simulink library "mbd_s32k11_ec_toolbox"  (Simulink 9.0)
settings: Solver=FixedStepDiscrete  StartTime=0.0  StopTime=10.0  FixedStep=0.1  RelTol=1e-3
InitFcn:
  | mbd_s32k11_consistency_checks(bdroot(gcs));
(part 1 of 2)
settings Model: Creator=evarshavskaya  LastModifiedBy=nxf30742

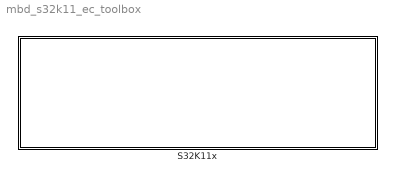
== system mbd_s32k11_ec_toolbox ==
  S32K11x : Subsystem

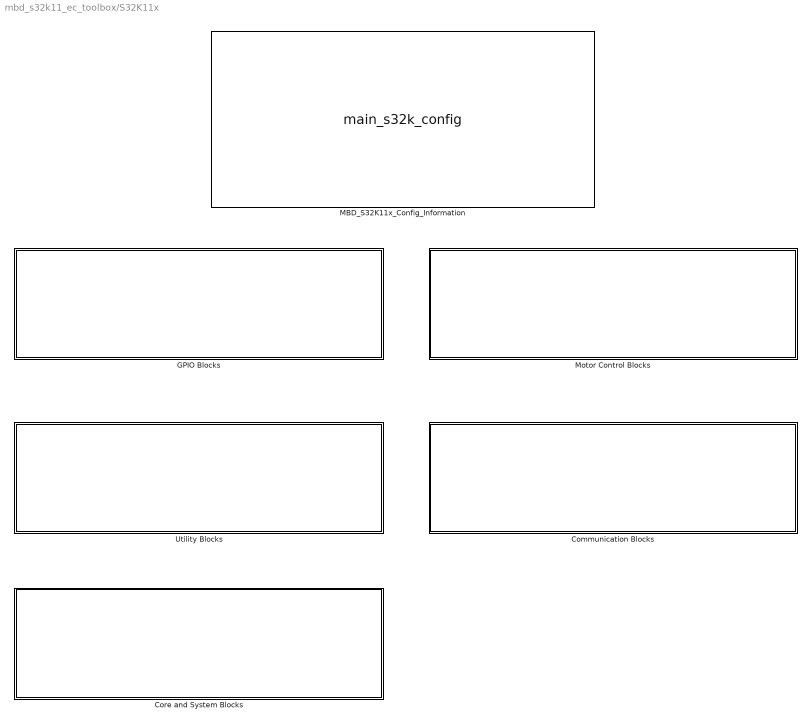
== system mbd_s32k11_ec_toolbox/S32K11x ==
  Communication Blocks : Subsystem
  Core and System Blocks : Subsystem
  GPIO Blocks : Subsystem
  MBD_S32K11x_Config_Information : S-Function  LoadFcn=|  InitFcn=|  FunctionName=main_s32k_config  SFunctionDeploymentMode=off  EnableBusSupport=off  mask(MBDTBX_EC_S32K11){disp_str=|, config_params=[], mcu_target_name=S32K116, mcu_target_package=48-LQFP, mcu_target_sram_size=17KB, mcu_system_clock_freq=40, mcu_xtal_freq=External 40, mcu_steptick_timer=LPIT Channel 0, mcu_steptick_prio=3, ds_import_enable=on, target_compiler=GCC, target_memory=FLASH, gcc_target_compile_opts=-mthumb -O1 -g -gstrict-dwarf, gcc_target_assemble_opts=-mthumb -g, gcc_target_link_opts=-mthumb, gcc_target_lib_opts=, gcc_target_default_lcf=on, gcc_target_user_lcf=S32K116_17_flash.ld, ghs_target_compile_opts=-thumb -fsingle -Ogeneral -Wundef -Wimplicit-int -Wshadow -Wtrigraphs --no_commons --gnu_asm -gnu99 -gdwarf-2 -G, ghs_target_assemble_opts=-thumb, ghs_target_link_opts=-thumb, ghs_target_lib_opts=, ghs_target_default_lcf=on, ghs_target_user_lcf=S32K116_17_flash.ld, iar_target_compile_opts=--thumb -Ol -e --debug --dlib_config normal, iar_target_assemble_opts=--thumb, iar_target_link_opts=--no_exceptions --vfe --inline, iar_target_lib_opts=, iar_target_default_lcf=on, iar_target_user_lcf=S32K116_17_flash.icf, pil_download_enable=off, rbl_download_enable=off, rbl_start_delay=5000, rbl_download_interface=OpenSDA, rbl_restart_request=off, rbl_com_port=Custom, rbl_com_port_custom=COM1, pil_download_rate=57600, pil_opensda_drive=Custom, pil_opensda_drive_custom=D, FTM_PWM_PcrCheckEnDis=on, FTM_Input_Edge_Inputs_PcrCheckEnDis=on, FTM_Dual_Edge_Inputs_PcrCheckEnDis=on, FTM_Quadrature_Inputs_PcrCheckEnDis=on, LPTMR_PcrCheckEnDis=on, PIT_PcrCheckEnDis=on, RTC_PcrCheckEnDis=on, FlexCAN_PcrCheckEnDis=on, FlexIO_PcrCheckEnDis=on, LPI2C_PcrCheckEnDis=on, LPSPI_PcrCheckEnDis=on, LPUART_PcrCheckEnDis=on, CMP_PcrCheckEnDis=on, GPIO_OutputPcrCheckEnDis=on, GPIO_InputPcrCheckEnDis=on, SBC_PcrCheckEnDis=on, AMMCLIB_PcrCheckEnDis=on, FM_PcrCheckEnDis=on, Profile_PcrCheckEnDis=on, ConfigParams_PcrCheckEnDis=on, ModelRef_PcrCheckEnDis=on, PDB0_PcrCheckEnDis=on, CSEc_PcrCheckEnDis=on, eDMA_PcrCheckEnDis=on, ADC_PcrCheckEnDis=on, WDOG_PcrCheckEnDis=on}
      LoadFcn=|
      | mbd_s32k_set_cur_model(bdroot(gcs));
      | mbd_s32k_block_load(bdroot(gcs));
      InitFcn=|
      | mbd_s32k_set_cur_model(bdroot(gcs)); 
      | mbd_s32k_update_model('init');       
      | mbd_s32k_check('MBDTBX_EC_S32K11');
      mask disp_str=|
      | Target : S32K144-64KB_SRAM
      | Package : 100-pin
      | System clock : 80 MHz
      | XTAL clock : External 8 MHz
      | Compiler : IAR
      | Target Type : FLASH
      | Download Code after build : off
      | Step Tick Interrupt Priority : 15
      mask prompts: disp_str "display_string"; mcu_target_name "Family"; mcu_target_package "Package"; mcu_target_sram_size "SRAM"; mcu_system_clock_freq "Clock Frequency MHz"; mcu_xtal_freq "XTAL Frequency MHz"; mcu_steptick_timer "Timer"; mcu_steptick_prio "Priority"; ds_import_enable "Generate S32 Design Studio ProjectInfo.xml file"; target_compiler "Compiler"; target_memory "Target Memory Model"; gcc_target_compile_opts "Compile Options"; gcc_target_assemble_opts "Assemble Options"; gcc_target_link_opts "Link Options"; gcc_target_lib_opts "Library Options"; gcc_target_default_lcf "Default Target Memory Definitions"; gcc_target_user_lcf "User Defined Target Memory Definitions"; ghs_target_compile_opts "Compile Options"; ghs_target_assemble_opts "Assemble Options"; ghs_target_link_opts "Link Options"; ghs_target_lib_opts "Library Options"; ghs_target_default_lcf "Default Target Memory Definitions"; ghs_target_user_lcf "User Defined Target Memory Definitions"; iar_target_compile_opts "Compile Options"; iar_target_assemble_opts "Assemble Options"; iar_target_link_opts "Link Options"; iar_target_lib_opts "Library Options"; iar_target_default_lcf "Default Target Memory Definitions"; iar_target_user_lcf "User Defined Target Memory Definitions"; pil_download_enable "Processor-in-the-Loop (PIL) Mode Download"; rbl_download_enable "Download Code after Build"; rbl_start_delay "Delay before start of application (ms)"; rbl_download_interface "Download Interface"; rbl_restart_request "Boot Assist Module (BAM) Restart Request"; rbl_com_port "COM Port"; rbl_com_port_custom "Custom COM Port"; pil_download_rate "Baud Rate"; pil_opensda_drive "OpenSDA Drive Name"; pil_opensda_drive_custom "Custom OpenSDA Drive Name"; FTM_PWM_PcrCheckEnDis "FTM PWM Config"; FTM_Input_Edge_Inputs_PcrCheckEnDis "FTM Input Edge Inputs"; FTM_Dual_Edge_Inputs_PcrCheckEnDis "FTM Dual Edge Inputs"; FTM_Quadrature_Inputs_PcrCheckEnDis "FTM Quadrature Inputs"; LPTMR_PcrCheckEnDis "LPTMR"; PIT_PcrCheckEnDis "PIT"; RTC_PcrCheckEnDis "RTC"; FlexCAN_PcrCheckEnDis "FlexCAN"; FlexIO_PcrCheckEnDis "FlexIO"; LPI2C_PcrCheckEnDis "LPI2C"; LPSPI_PcrCheckEnDis "LPSPI"; LPUART_PcrCheckEnDis "LPUART"; CMP_PcrCheckEnDis "CMP"; GPIO_OutputPcrCheckEnDis "GPIO Output"; GPIO_InputPcrCheckEnDis "GPIO Input"; SBC_PcrCheckEnDis "SBC"; AMMCLIB_PcrCheckEnDis "AMMCLIB"; FM_PcrCheckEnDis "FreeMaster"; Profile_PcrCheckEnDis "Profile"; ConfigParams_PcrCheckEnDis "Config Params"; ModelRef_PcrCheckEnDis "Model Reference"; PDB0_PcrCheckEnDis "PDB"; CSEc_PcrCheckEnDis "CSEc"; eDMA_PcrCheckEnDis "eDMA"; ADC_PcrCheckEnDis "ADC"; WDOG_PcrCheckEnDis "WDOG"
      mask help: Model-Based Design Toolbox Config block for S32K11x family of processors.
      mask init:
      | mbd_s32k_config_com_ports_cbk('populate_drop_down');
      | maskStr = mbd_s32k_mb_display_string();
      settings: NameChangeFcn=mbd_s32k_model_close;
      settings: CopyFcn=|
      | mbd_s32k_set_cur_model(bdroot(gcs));
      | mbd_s32k_check('MBDTBX_EC_S32K11');
      | mbd_s32k_update_model('copy');
      | set_param(gcb, 'mcu_target_name', 'S32K116');
      settings: ModelCloseFcn=|
      | mbd_s32k_set_cur_model(bdroot(gcs));
      | mbd_s32k_model_close;
      settings: CloseFcn=|
      | mbd_s32k_set_cur_model(bdroot(gcs));
      | mbd_s32k_check('MBDTBX_EC_S32K11');
      | mbd_s32k_update_model('copy');
      mask Help: web(fullfile(mbd_s32k14_block_help, 'main_config', 'main_config.html'));
      mask TypeOptions mcu_target_name: S32K116 | S32K118
      mask Callback mcu_target_name: mbd_s32k11_config_target_cbk('mcu_target_name')
      mask TypeOptions mcu_target_package: 48-LQFP | 32-QFN
      mask Callback mcu_target_package: mbd_s32k11_config_target_cbk('mcu_target_package')
      mask TypeOptions mcu_target_sram_size: 17KB
      mask Callback mcu_target_sram_size: mbd_s32k11_config_target_cbk('mcu_target_sram_size')
      mask TypeOptions mcu_system_clock_freq: 40
      mask TypeOptions mcu_xtal_freq: External 40
      mask TypeOptions mcu_steptick_timer: LPIT Channel 0 | Suppress
      mask TypeOptions mcu_steptick_prio: 0 | 1 | 2 | 3
      mask TypeOptions target_compiler: IAR | GCC | GreenHills Multi
      mask Callback target_compiler: mbd_s32k_config_compiler_cbk('target_compiler')
      mask TypeOptions target_memory: FLASH
      mask Callback target_memory:
      | mbd_s32k11_config_target_cbk('mcu_target_memory')
      | mbd_s32k_config_memory_cbk('target_memory')
      mask Callback gcc_target_default_lcf: mbd_s32k_config_lcf_cbk('gcc_target_default_lcf')
      mask TypeOptions gcc_target_user_lcf: S32K116_17_flash.ld | S32K116_17_flash_bam.ld
      mask Callback ghs_target_default_lcf: mbd_s32k_config_lcf_cbk('ghs_target_default_lcf')
      mask TypeOptions ghs_target_user_lcf: S32K116_17_flash.ld | S32K116_17_flash_bam.ld
      mask Callback iar_target_default_lcf: mbd_s32k_config_lcf_cbk('iar_target_default_lcf')
      mask TypeOptions iar_target_user_lcf: S32K116_17_flash.icf | S32K116_17_flash_bam.icf
      mask Callback pil_download_enable: mbd_s32k_config_pil_cbk('pil_download_enable')
      mask Callback rbl_download_enable: mbd_s32k_config_pil_cbk('rbl_download_enable');
      mask TypeOptions rbl_download_interface: Serial | OpenSDA
      mask Callback rbl_download_interface: mbd_s32k_config_pil_cbk('rbl_download_interface')
      mask TypeOptions rbl_com_port: COM1 | Custom
      mask Callback rbl_com_port: mbd_s32k_config_com_ports_cbk('populate_drop_down')
      mask TypeOptions pil_download_rate: 9600 | 14400 | 19200 | 38400 | 56000 | 57600 | 115200
      mask TypeOptions pil_opensda_drive: Custom
      mask Callback pil_opensda_drive:
      | mbd_s32k_config_vol_disks_cbk('populate_drop_down');
      | mbd_s32k_config_vol_disks_cbk('enable_custom');
      mask DialogControl rbl_com_button Prompt: Refresh
      mask DialogControl rbl_com_button Callback: mbd_s32k_config_com_ports_cbk('populate_drop_down')
      mask DialogControl pil_opensda_refresh Prompt: Refresh
      mask DialogControl pil_opensda_refresh Callback: mbd_s32k_config_vol_disks_cbk('populate_drop_down')
      mask DialogControl Container17 Prompt: Consistency checks
      mask Display: disp(maskStr);
  Motor Control Blocks : Subsystem
  Utility Blocks : Subsystem

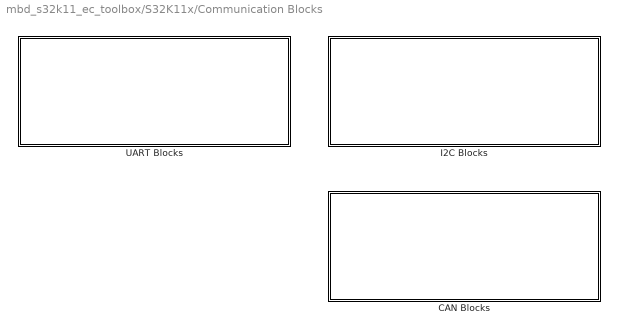
== system mbd_s32k11_ec_toolbox/S32K11x/Communication Blocks ==
  CAN Blocks : Subsystem
  I2C Blocks : Subsystem
  UART Blocks : Subsystem

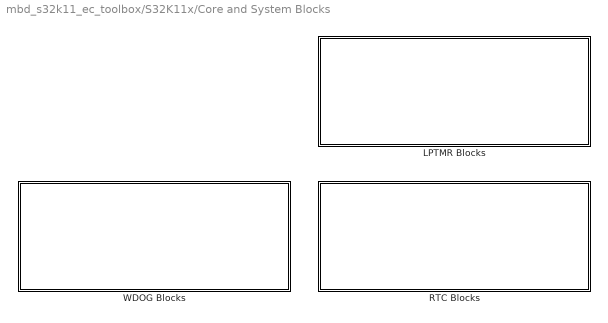
== system mbd_s32k11_ec_toolbox/S32K11x/Core and System Blocks ==
  LPTMR Blocks : Subsystem
  RTC Blocks : Subsystem
  WDOG Blocks : Subsystem

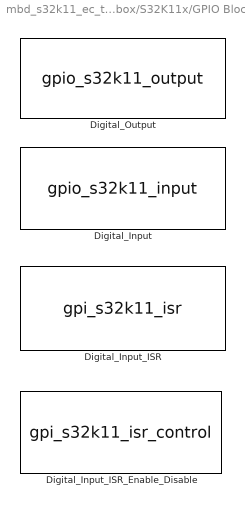
== system mbd_s32k11_ec_toolbox/S32K11x/GPIO Blocks ==
  Digital_Input : S-Function  FunctionName=gpio_s32k11_input  SFunctionDeploymentMode=off  EnableBusSupport=off  mask(gpio_s32k11_input){gpio_pin=PTA0: [PTA0 | Port A I/O], pull_resistor=None, passive_filter=off}
      mask prompts: gpio_pin "Input Pin"; pull_resistor "Pull Resistor Select"; passive_filter "Passive Filter Enable"
      mask help: Select a General Purpose Input Pin as a Source.
      mask init:
      | mbd_s32k_gpi_init;
      settings: NameChangeFcn=mbd_s32k_name_check (gcb);
      mask Help: web(fullfile(mbd_s32k14_block_help, 'gpio', 'gpio_input.html'));
      mask TypeOptions gpio_pin: PTA0: [PTA0 | Port A I/O] | PTA1: [PTA1 | Port A I/O] | PTA2: [PTA2 | Port A I/O] | PTA3: [PTA3 | Port A I/O] | PTA4: [PTA4 | Port A I/O] | PTA5: [PTA5 | Port A I/O] | PTA7: [PTA7 | Port A I/O] | PTA10: [PTA10 | Port A I/O] | PTA11: [PTA11 | Port A I/O] | PTA12: [PTA12 | Port A I/O] | PTA13: [PTA13 | Port A I/O] | PTB0: [PTB0 | Port B I/O] | PTB1: [PTB1 | Port B I/O] | PTB2: [PTB2 | Port B I/O] | PTB3: [PTB3 | Port B I/O] | PTB4: [PTB4 | Port B I/O] | PTB5: [PTB5 | Port B I/O] | PTB6: [PTB6 | Port B I/O] | PTB7: [PTB7 | Port B I/O] | PTB13: [PTB13 | Port B I/O] | PTC1: [PTC1 | Port C I/O] | PTC2: [PTC2 | Port C I/O] | PTC3: [PTC3 | Port C I/O] | PTC4: [PTC4 | Port C I/O] | PTC5: [PTC5 | Port C I/O] | PTC6: [PTC6 | Port C I/O] | PTC7: [PTC7 | Port C I/O] | PTC8: [PTC8 | Port C I/O] | PTC9: [PTC9 | Port C I/O] | PTC14: [PTC14 | Port C I/O] | PTC15: [PTC15 | Port C I/O] | PTC16: [PTC16 | Port C I/O] | PTD0: [PTD0 | Port D I/O] | PTD1: [PTD1 | Port D I/O] | PTD2: [PTD2 | Port D I/O] | PTD3: [PTD3 | Port D I/O] | PTD5: [PTD5 | Port D I/O] | PTD15: [PTD15 | Port D I/O] | PTD16: [PTD16 | Port D I/O] | PTE4: [PTE4 | Port E I/O] | PTE5: [PTE5 | Port E I/O] | PTE8: [PTE8 | Port E I/O] | PTE9: [PTE9 | Port E I/O]
      mask Callback gpio_pin: mbd_s32k_display_pin_info('gpio', gcb, 'gpio_pin')
      mask TypeOptions pull_resistor: None | Pulldown | Pullup
      mask Display:
      | port_label('output',1,'input');
      | disp(maskStr);
  Digital_Input_ISR : S-Function  FunctionName=gpi_s32k11_isr  SFunctionDeploymentMode=off  EnableBusSupport=off  mask(gpi_s32k11_isr){gpio_pin=PTA0: [PTA0 | Port A I/O], irqc=when logic 0, prio=0}
      mask prompts: gpio_pin "Input Pin"; irqc "Interrupt Configuration"; prio "ISR Priority (0 to 3)"
      mask help: Configure a General Purpose Input Pin to generate an ISR.
      mask init:
      | mbd_s32k_gpi_isr_init;
      settings: NameChangeFcn=mbd_s32k_name_check (gcb);
      mask Help: web(fullfile(mbd_s32k11_block_help, 'gpio', 'gpi_isr.html'));
      mask TypeOptions gpio_pin: PTA0: [PTA0 | Port A I/O] | PTA1: [PTA1 | Port A I/O] | PTA2: [PTA2 | Port A I/O] | PTA3: [PTA3 | Port A I/O] | PTA4: [PTA4 | Port A I/O] | PTA5: [PTA5 | Port A I/O] | PTA7: [PTA7 | Port A I/O] | PTA10: [PTA10 | Port A I/O] | PTA11: [PTA11 | Port A I/O] | PTA12: [PTA12 | Port A I/O] | PTA13: [PTA13 | Port A I/O] | PTB0: [PTB0 | Port B I/O] | PTB1: [PTB1 | Port B I/O] | PTB2: [PTB2 | Port B I/O] | PTB3: [PTB3 | Port B I/O] | PTB4: [PTB4 | Port B I/O] | PTB5: [PTB5 | Port B I/O] | PTB6: [PTB6 | Port B I/O] | PTB7: [PTB7 | Port B I/O] | PTB13: [PTB13 | Port B I/O] | PTC1: [PTC1 | Port C I/O] | PTC2: [PTC2 | Port C I/O] | PTC3: [PTC3 | Port C I/O] | PTC4: [PTC4 | Port C I/O] | PTC5: [PTC5 | Port C I/O] | PTC6: [PTC6 | Port C I/O] | PTC7: [PTC7 | Port C I/O] | PTC8: [PTC8 | Port C I/O] | PTC9: [PTC9 | Port C I/O] | PTC14: [PTC14 | Port C I/O] | PTC15: [PTC15 | Port C I/O] | PTC16: [PTC16 | Port C I/O] | PTD0: [PTD0 | Port D I/O] | PTD1: [PTD1 | Port D I/O] | PTD2: [PTD2 | Port D I/O] | PTD3: [PTD3 | Port D I/O] | PTD5: [PTD5 | Port D I/O] | PTD15: [PTD15 | Port D I/O] | PTD16: [PTD16 | Port D I/O] | PTE4: [PTE4 | Port E I/O] | PTE5: [PTE5 | Port E I/O] | PTE8: [PTE8 | Port E I/O] | PTE9: [PTE9 | Port E I/O]
      mask Callback gpio_pin: mbd_s32k_display_pin_info('gpio', gcb, 'gpio_pin')
      mask TypeOptions irqc: when logic 0 | on rising-edge | on falling-edge | on either-edge | when logic 1
      mask TypeOptions prio: 0 | 1 | 2 | 3
      mask Display:
      | port_label('output',1,'function');
      | disp(maskStr);
  Digital_Input_ISR_Enable_Disable : S-Function  FunctionName=gpi_s32k11_isr_control  SFunctionDeploymentMode=off  EnableBusSupport=off  mask(gpi_s32k11_isr_control){gpio_pin=PTA0: [PTA0 | Port A I/O], irqc=request disabled}
      mask prompts: gpio_pin "Input Pin"; irqc "Interrupt Configuration"
      mask help: This block enables or disables the interrupt for GPI ISR block.
      mask init:
      | mbd_s32k_gpi_isr_control_init;
      settings: NameChangeFcn=mbd_s32k_name_check(gcb);
      mask Help: web(fullfile(mbd_s32k11_block_help, 'gpio', 'gpi_isr_control.html'));
      mask TypeOptions gpio_pin: PTA0: [PTA0 | Port A I/O] | PTA1: [PTA1 | Port A I/O] | PTA2: [PTA2 | Port A I/O] | PTA3: [PTA3 | Port A I/O] | PTA4: [PTA4 | Port A I/O] | PTA5: [PTA5 | Port A I/O] | PTA7: [PTA7 | Port A I/O] | PTA10: [PTA10 | Port A I/O] | PTA11: [PTA11 | Port A I/O] | PTA12: [PTA12 | Port A I/O] | PTA13: [PTA13 | Port A I/O] | PTB0: [PTB0 | Port B I/O] | PTB1: [PTB1 | Port B I/O] | PTB2: [PTB2 | Port B I/O] | PTB3: [PTB3 | Port B I/O] | PTB4: [PTB4 | Port B I/O] | PTB5: [PTB5 | Port B I/O] | PTB6: [PTB6 | Port B I/O] | PTB7: [PTB7 | Port B I/O] | PTB13: [PTB13 | Port B I/O] | PTC1: [PTC1 | Port C I/O] | PTC2: [PTC2 | Port C I/O] | PTC3: [PTC3 | Port C I/O] | PTC4: [PTC4 | Port C I/O] | PTC5: [PTC5 | Port C I/O] | PTC6: [PTC6 | Port C I/O] | PTC7: [PTC7 | Port C I/O] | PTC8: [PTC8 | Port C I/O] | PTC9: [PTC9 | Port C I/O] | PTC14: [PTC14 | Port C I/O] | PTC15: [PTC15 | Port C I/O] | PTC16: [PTC16 | Port C I/O] | PTD0: [PTD0 | Port D I/O] | PTD1: [PTD1 | Port D I/O] | PTD2: [PTD2 | Port D I/O] | PTD3: [PTD3 | Port D I/O] | PTD5: [PTD5 | Port D I/O] | PTD15: [PTD15 | Port D I/O] | PTD16: [PTD16 | Port D I/O] | PTE4: [PTE4 | Port E I/O] | PTE5: [PTE5 | Port E I/O] | PTE8: [PTE8 | Port E I/O] | PTE9: [PTE9 | Port E I/O]
      mask Callback gpio_pin: mbd_s32k_display_pin_info('gpio', gcb, 'gpio_pin')
      mask TypeOptions irqc: request disabled | when logic 0 | on rising-edge | on falling-edge | on either-edge | when logic 1
      mask Display: disp(maskStr)
  Digital_Output : S-Function  FunctionName=gpio_s32k11_output  SFunctionDeploymentMode=off  EnableBusSupport=off  mask(gpio_s32k11_output){gpio_pin=PTA0: [PTA0 | Port A I/O], drive_strength=Low}
      mask prompts: gpio_pin "Output Pin"; drive_strength "Drive Strength"
      mask help: Select a General Purpose Output Pin as a Sink.
      mask init:
      | mbd_s32k_gpo_init;
      settings: NameChangeFcn=mbd_s32k_name_check (gcb);
      mask Help: web(fullfile(mbd_s32k11_block_help, 'gpio', 'gpio_output.html'));
      mask TypeOptions gpio_pin: PTA0: [PTA0 | Port A I/O] | PTA1: [PTA1 | Port A I/O] | PTA2: [PTA2 | Port A I/O] | PTA3: [PTA3 | Port A I/O] | PTA4: [PTA4 | Port A I/O] | PTA5: [PTA5 | Port A I/O] | PTA7: [PTA7 | Port A I/O] | PTA10: [PTA10 | Port A I/O] | PTA11: [PTA11 | Port A I/O] | PTA12: [PTA12 | Port A I/O] | PTA13: [PTA13 | Port A I/O] | PTB0: [PTB0 | Port B I/O] | PTB1: [PTB1 | Port B I/O] | PTB2: [PTB2 | Port B I/O] | PTB3: [PTB3 | Port B I/O] | PTB4: [PTB4 | Port B I/O] | PTB5: [PTB5 | Port B I/O] | PTB6: [PTB6 | Port B I/O] | PTB7: [PTB7 | Port B I/O] | PTB13: [PTB13 | Port B I/O] | PTC1: [PTC1 | Port C I/O] | PTC2: [PTC2 | Port C I/O] | PTC3: [PTC3 | Port C I/O] | PTC4: [PTC4 | Port C I/O] | PTC5: [PTC5 | Port C I/O] | PTC6: [PTC6 | Port C I/O] | PTC7: [PTC7 | Port C I/O] | PTC8: [PTC8 | Port C I/O] | PTC9: [PTC9 | Port C I/O] | PTC14: [PTC14 | Port C I/O] | PTC15: [PTC15 | Port C I/O] | PTC16: [PTC16 | Port C I/O] | PTD0: [PTD0 | Port D I/O] | PTD1: [PTD1 | Port D I/O] | PTD2: [PTD2 | Port D I/O] | PTD3: [PTD3 | Port D I/O] | PTD5: [PTD5 | Port D I/O] | PTD15: [PTD15 | Port D I/O] | PTD16: [PTD16 | Port D I/O] | PTE4: [PTE4 | Port E I/O] | PTE5: [PTE5 | Port E I/O] | PTE8: [PTE8 | Port E I/O] | PTE9: [PTE9 | Port E I/O]
      mask Callback gpio_pin: mbd_s32k_display_pin_info('gpio', gcb, 'gpio_pin')
      mask TypeOptions drive_strength: Low | High
      mask Display:
      | disp(st);
      | port_label('input',1,'output')

== system mbd_s32k11_ec_toolbox/S32K11x/Motor Control Blocks ==
  CMP Blocks : Subsystem

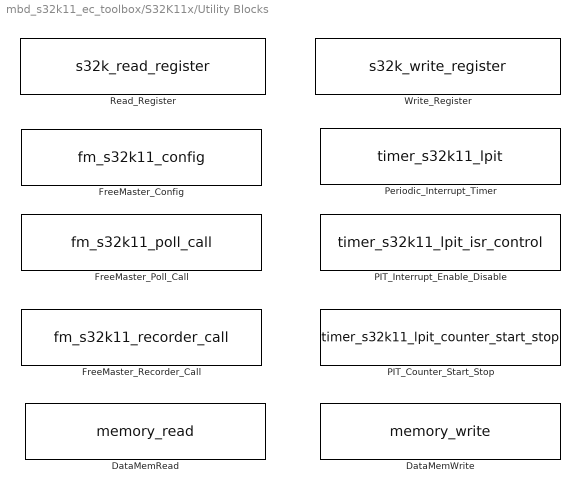
== system mbd_s32k11_ec_toolbox/S32K11x/Utility Blocks ==
  DataMemRead : S-Function  FunctionName=memory_read  Parameters=ptr_type  SFunctionDeploymentMode=off  EnableBusSupport=off  mask(memory_read){base=0x20000000, offset=0x0000, ptr=uint32_t}
      mask prompts: base "Enter base address (e.f...0x20000000)"; offset "Enter Offset from base Address (e.g. ..0x4)"; ptr "Pointer type"
      mask help: This block provides direct access to memory by address and offset into any memory section the processor has access. This block provides a direct memory read from the specified memory location.
      mask init:
      | [maskStr, ptr_type] = mbd_s32k_mem_init();
      settings: NameChangeFcn=mbd_s32k_name_check(gcb);
      mask Help: web(fullfile(mbd_s32k11_block_help, 'memory', 'memory_read.html'));
      mask Callback base:
      | str = get_param(gcb, 'base');
      | len = length(str);
      | size = 8;
      | 
      | if (len > 2)
      |     if (strcmp(str(1:2), '0x'))
      |         str = str(3:len);
      |     end
      | end
      | %check if str is a valid hex number. if not, make a valid hex
      | isAllHex = all(isstrprop(str, 'xdigit'));
      | if (~isAllHex)
      |         str = dec2hex(0,size);
      |         len = length(str);
      | end
      | %get address from string
      | value = hex2dec(str);
      | 
      | %check range
      | if (value < 0)
      |     value = 0;
      | elseif (value > hex2dec('FFFF0000'))
      |     value = hex2dec('FFFF0000');
      | end
      | 
      | set_param(gcb, 'base', strcat('0x',dec2hex(value,size)));
      mask Callback offset:
      | str = get_param(gcb, 'offset');
      | len = length(str);
      | size = 4;
      | 
      | if (len > 2)
      |     if (strcmp(str(1:2), '0x'))
      |         str = str(3:len);
      |     end
      | end
      | %check if str is a valid hex number. if not, make a valid hex
      | isAllHex = all(isstrprop(str, 'xdigit'));
      | if (~isAllHex)
      |         str = dec2hex(0,size);
      |         len = length(str);
      | end
      | %get address from string
      | value = hex2dec(str);
      | 
      | %check range
      | if (value < 0)
      |     value = 0;
      | elseif (value > hex2dec('FFFF'))
      |     value = hex2dec('FFFF');
      | end
      | 
      | set_param(gcb, 'offset', strcat('0x',dec2hex(value,size)));
      mask TypeOptions ptr: uint8_t | uint16_t | uint32_t
      mask Display:
      | port_label('output',1,'Output Signal');
      | 
      | disp(maskStr);
  DataMemWrite : S-Function  FunctionName=memory_write  Parameters=ptr_type  SFunctionDeploymentMode=off  EnableBusSupport=off  mask(memory_write){base=0x20000000, offset=0x0000, ptr=uint32_t}
      mask prompts: base "Enter base address (e.g. 0x20000000)"; offset "Enter Offset from base Address (e.g. 0x4)"; ptr "Pointer type"
      mask help: This block provides direct access to memory by address and offset into any memory section the processor has access. This block allows a direct write to the specified memory location.
      mask init:
      | [maskStr, ptr_type] = mbd_s32k_mem_init();
      settings: NameChangeFcn=mbd_s32k_name_check(gcb);
      mask Help: web(fullfile(mbd_s32k11_block_help, 'memory', 'memory_write.html'));
      mask Callback base:
      | str = get_param(gcb, 'base');
      | len = length(str);
      | size = 8;
      | 
      | if (len > 2)
      |     if (strcmp(str(1:2), '0x'))
      |         str = str(3:len);
      |     end
      | end
      | %check if str is a valid hex number. if not, make a valid hex
      | isAllHex = all(isstrprop(str, 'xdigit'));
      | if (~isAllHex)
      |         str = dec2hex(0,size);
      |         len = length(str);
      | end
      | %get address from string
      | value = hex2dec(str);
      | 
      | %check range
      | if (value < 0)
      |     value = 0;
      | elseif (value > hex2dec('FFFF0000'))
      |     value = hex2dec('FFFF0000');
      | end
      | 
      | set_param(gcb, 'base', strcat('0x',dec2hex(value,size)));
      mask Callback offset:
      | str = get_param(gcb, 'offset');
      | len = length(str);
      | size = 4;
      | 
      | if (len > 2)
      |     if (strcmp(str(1:2), '0x'))
      |         str = str(3:len);
      |     end
      | end
      | %check if str is a valid hex number. if not, make a valid hex
      | isAllHex = all(isstrprop(str, 'xdigit'));
      | if (~isAllHex)
      |         str = dec2hex(0,size);
      |         len = length(str);
      | end
      | %get address from string
      | value = hex2dec(str);
      | 
      | %check range
      | if (value < 0)
      |     value = 0;
      | elseif (value > hex2dec('FFFF'))
      |     value = hex2dec('FFFF');
      | end
      | 
      | set_param(gcb, 'offset', strcat('0x',dec2hex(value,size)));
      mask TypeOptions ptr: uint8_t | uint16_t | uint32_t
      mask Display:
      | port_label('input',1,'Input Signal');
      | 
      | disp(maskStr);
  FreeMaster_Config : S-Function  FunctionName=fm_s32k11_config  Parameters=sFuncParams  SFunctionDeploymentMode=off  EnableBusSupport=off  mask(fm_s32k11_config){interface=LPUART0, baudrate=115200, rxd=PTA2: [LPUART0_RX | Receive], txd=PTA3: [LPUART0_TX | Transmit], mode=Poll-driven, isr_prio=0, show_adv_opts=off, use_scope=on, max_scope_vars=8, use_recorder=on, max_rec_vars=8, rec_buff_size=1024, rec_timebase=0, rec_timebase_unit=seconds, comm_buffer_size_auto=on, comm_buffer_size=255, comm_rqueue_size_default=on, comm_rqueue_size=32}
      mask prompts: baudrate "Baud Rate"; rxd "RxD pin"; txd "TxD pin"; isr_prio "ISR Priority"; show_adv_opts "Show Advanced Options"; use_scope "Use Scope"; max_scope_vars "Max Variables"; use_recorder "Use Reccorder"; max_rec_vars "Max Variables"; rec_buff_size "Buffer size (0 - 65536)"; rec_timebase "Timebase (0 - 16384)"; comm_buffer_size_auto "Automatic buffer size"; comm_buffer_size "Buffer size (1-255)"; comm_rqueue_size_default "Default FIFO receiver queue size"; comm_rqueue_size "FIFO receiver queue size (1 - 255)"
      mask help: This block allows the user to configure the FreeMaster embedded-side software driver.
      mask init:
      | mbd_s32k_fm_config_init;
      | mbd_s32k_fm_display_instances;
      settings: NameChangeFcn=mbd_s32k_name_check(gcb);
      mask Help: web(fullfile(mbd_s32k14_block_help, 'fm', 'fm_config.html'));
      mask TypeOptions interface: LPUART0 | LPUART1 | CAN0
      mask Callback interface:
      | mbd_s32k_fm_config_cbk('interface');
      | mbd_s32k_fm_display_instances();
      mask TypeOptions baudrate: 1200 | 2400 | 4800 | 9600 | 14400 | 19200 | 38400 | 56000 | 57600 | 115200 | 128000 | 256000
      mask TypeOptions rxd: PTA2: [LPUART0_RX | Receive] | PTB0: [LPUART0_RX | Receive] | PTC2: [LPUART0_RX | Receive]
      mask TypeOptions txd: PTA3: [LPUART0_TX | Transmit] | PTB1: [LPUART0_TX | Transmit] | PTC3: [LPUART0_TX | Transmit]
      mask TypeOptions mode: Long Interrupt | Short Interrupt | Poll-driven
      mask Callback mode: mbd_s32k_fm_config_cbk('mode')
      mask TypeOptions isr_prio: 0 | 1 | 2 | 3
      mask Callback show_adv_opts: mbd_s32k_fm_config_cbk('show_adv_opts')
      mask Callback use_scope: mbd_s32k_fm_config_cbk('use_scope')
      mask TypeOptions max_scope_vars: 2 | 3 | 4 | 5 | 6 | 7 | 8
      mask Callback use_recorder: mbd_s32k_fm_config_cbk('use_recorder')
      mask TypeOptions max_rec_vars: 2 | 3 | 4 | 5 | 6 | 7 | 8
      mask TypeOptions rec_timebase_unit: seconds | milliseconds | microseconds | nanoseconds
      mask Callback comm_buffer_size_auto: mbd_s32k_fm_config_cbk('comm_buffer_size_auto')
      mask Callback comm_rqueue_size_default: mbd_s32k_fm_config_cbk('comm_rqueue_size_default')
      mask Display: disp(maskStr)
  FreeMaster_Poll_Call : S-Function  FunctionName=fm_s32k11_poll_call  SFunctionDeploymentMode=off  EnableBusSupport=off  mask(fm_s32k11_poll_call){}
      mask help: This block allows the user to call the FMSTR_Call function in other places then main loop. The FMSTR_Call is placed in the main application loop when this block is not used.
      settings: NameChangeFcn=mbd_s32k_name_check(gcb);
      mask Help: web(fullfile(mbd_s32k14_block_help, 'fm', 'fm_poll_call.html'));
      mask Display: disp('FreeMaster Poll Call')
  FreeMaster_Recorder_Call : S-Function  FunctionName=fm_s32k11_recorder_call  SFunctionDeploymentMode=off  EnableBusSupport=off  mask(fm_s32k11_recorder_call){}
      mask help: This block allows the user to call the FMSTR_Recorder function periodically, in places where the data recording should occur.
      settings: NameChangeFcn=mbd_s32k_name_check(gcb);
      mask Help: web(fullfile(mbd_s32k14_block_help, 'fm', 'fm_recorder_call.html'));
      mask Display: disp('FreeMaster Recorder Call')
  PIT_Counter_Start_Stop : S-Function  FunctionName=timer_s32k11_lpit_counter_start_stop  SFunctionDeploymentMode=off  EnableBusSupport=off  mask(timer_s32k11_lpit_counter_start_stop){channel=1, action=Start}
      mask prompts: channel "PIT channel"
      mask help: This block starts or stops the timer channel for PIT block.
      mask init:
      | maskStr = mbd_s32k_lpit_start_stop_init();
      settings: NameChangeFcn=mbd_s32k_name_check(gcb);
      mask Help: web(fullfile(mbd_s32k11_block_help, 'lpit', 'timer_lpit_counter_start_stop.html'));
      mask TypeOptions channel: 0 | 1 | 2 | 3
      mask TypeOptions action: Start | Stop
      mask Display: disp(maskStr)
  PIT_Interrupt_Enable_Disable : S-Function  FunctionName=timer_s32k11_lpit_isr_control  SFunctionDeploymentMode=off  EnableBusSupport=off  mask(timer_s32k11_lpit_isr_control){channel=1, enable=off}
      mask prompts: channel "PIT channel"; enable "Enable Timer Interrupt"
      mask help: This block enables or disables the interrupt for PIT block.
      mask init:
      | maskStr = mbd_s32k_lpit_disen_init();
      settings: NameChangeFcn=mbd_s32k_name_check(gcb);
      mask Help: web(fullfile(mbd_s32k11_block_help, 'lpit', 'timer_lpit_isr_control.html'));
      mask TypeOptions channel: 0 | 1 | 2 | 3
      mask Display: disp(maskStr)
  Periodic_Interrupt_Timer : S-Function  FunctionName=timer_s32k11_lpit  SFunctionDeploymentMode=off  EnableBusSupport=off  mask(timer_s32k11_lpit){channel=1, period=500000, prio=15, startCounter=on}
      mask prompts: channel "PIT Channel"; period "Period Value (us)"; prio "ISR Priority (0 to 15)"; startCounter "Start counter immediately after initialization"
      mask help: This block triggers an interrupt routine to execute every timeout of this LPIT channel in 32-bit Periodic Counter Mode.
      mask init:
      | maskStr = mbd_s32k_lpit_init();
      settings: NameChangeFcn=mbd_s32k_name_check(gcb);
      mask Help: web(fullfile(mbd_s32k11_block_help, 'lpit', 'timer_pit.html'));
      mask TypeOptions channel: 0 | 1 | 2 | 3
      mask TypeOptions prio: 0 | 1 | 2 | 3 | 4 | 5 | 6 | 7 | 8 | 9 | 10 | 11 | 12 | 13 | 14 | 15
      mask Display:
      | disp(maskStr)
      | port_label('output',1,'trigger')
  Read_Register : S-Function  FunctionName=s32k_read_register  Parameters=index  SFunctionDeploymentMode=off  EnableBusSupport=off  mask(Read_Register){periph=ADC0, reg=SC1A, addr=0x4003B000, regSize=32, pcc_clock=ADC0_CLK}
      mask prompts: periph "Peripheral"; reg "Register"; addr "Address"; regSize "Size (bits)"; pcc_clock "PCC Clock"
      mask help: This block allows direct access to read a register.
      mask init:
      | mbd_s32k_rw_register_init;
      mask Help: web(fullfile(mbd_s32k11_block_help, 'reg', 'read_register.html'));
      mask TypeOptions periph: ADC0 | AIPS | CAN0 | CMP0 | CMU_FC_0 | CMU_FC_1 | CRC | CSE_PRAM | DMA | DMAMUX | EIM | ERM | FLEXIO | FTFC | FTM0 | FTM1 | LMEM | LPI2C0 | LPIT0 | LPSPI0 | LPTMR0 | LPUART0 | LPUART1 | MCM | MPU | MSCM | MTB_DWT | PCC | PDB0 | PMC | PORTA | PORTB | PORTC | PORTD | PORTE | PTA | PTB | PTC | PTD | PTE | RCM | RTC | S32_NVIC | S32_SCB | S32_SysTick | SCG | SIM | SMC | TRGMUX | WDOG
      mask Callback periph: mbd_s32k_periph_update_cbk('read');
      mask TypeOptions reg: SC1A | SC1B | SC1C | SC1D | SC1E | SC1F | SC1G | SC1H | SC1I | SC1J | SC1K | SC1L | SC1M | SC1N | SC1O | SC1P | CFG1 | CFG2 | RA | RB | RC | RD | RE | RF | RG | RH | RI | RJ | RK | RL | RM | RN | RO | RP | CV1 | CV2 | SC2 | SC3 | BASE_OFS | OFS | USR_OFS | XOFS | YOFS | G | UG | CLPS | CLP3 | CLP2 | CLP1 | CLP0 | CLPX | CLP9 | CLPS_OFS | CLP3_OFS | CLP2_OFS | CLP1_OFS | CLP0_OFS | CLPX_OFS | CLP9_OFS
      mask Callback reg: mbd_s32k_reg_update_cbk;
      mask DialogControl descript Prompt: ADC Status and Control Register 1
      mask Display:
      | port_label('output',1,'Output');
      | disp(maskStr);
  Write_Register : S-Function  FunctionName=s32k_write_register  Parameters=index  SFunctionDeploymentMode=off  EnableBusSupport=off  mask(Write_Register){periph=ADC0, reg=SC1A, addr=0x4003B000, regsize=32, pcc_clock=ADC0_CLK}
      mask prompts: periph "Peripheral"; reg "Register"; addr "Address"; regsize "Size (bits)"; pcc_clock "PCC clock"
      mask help: This block allows direct access to write a register
      mask init:
      | mbd_s32k_rw_register_init;
      mask Help: web(fullfile(mbd_s32k11_block_help, 'reg', 'write_register.html'));
      mask TypeOptions periph: ADC0 | AIPS | CAN0 | CMP0 | CMU_FC_0 | CMU_FC_1 | CRC | CSE_PRAM | DMA | DMAMUX | EIM | ERM | FLEXIO | FTFC | FTM0 | FTM1 | LMEM | LPI2C0 | LPIT0 | LPSPI0 | LPTMR0 | LPUART0 | LPUART1 | MCM | MPU | MSCM | MTB_DWT | PCC | PDB0 | PMC | PORTA | PORTB | PORTC | PORTD | PORTE | PTA | PTB | PTC | PTD | PTE | RCM | RTC | S32_NVIC | S32_SCB | S32_SysTick | SCG | SIM | SMC | TRGMUX | WDOG
      mask Callback periph: mbd_s32k_periph_update_cbk('write')
      mask TypeOptions reg: SC1A | SC1B | SC1C | SC1D | SC1E | SC1F | SC1G | SC1H | SC1I | SC1J | SC1K | SC1L | SC1M | SC1N | SC1O | SC1P | CFG1 | CFG2 | CV1 | CV2 | SC2 | SC3 | BASE_OFS | OFS | USR_OFS | XOFS | YOFS | G | UG | CLPS | CLP3 | CLP2 | CLP1 | CLP0 | CLPX | CLP9 | CLPS_OFS | CLP3_OFS | CLP2_OFS | CLP1_OFS | CLP0_OFS | CLPX_OFS | CLP9_OFS
      mask Callback reg: mbd_s32k_reg_update_cbk;
      mask DialogControl descript Prompt: ADC Status and Control Register 1
      mask Display:
      | port_label('input',1,'Input ');
      | disp(maskStr);

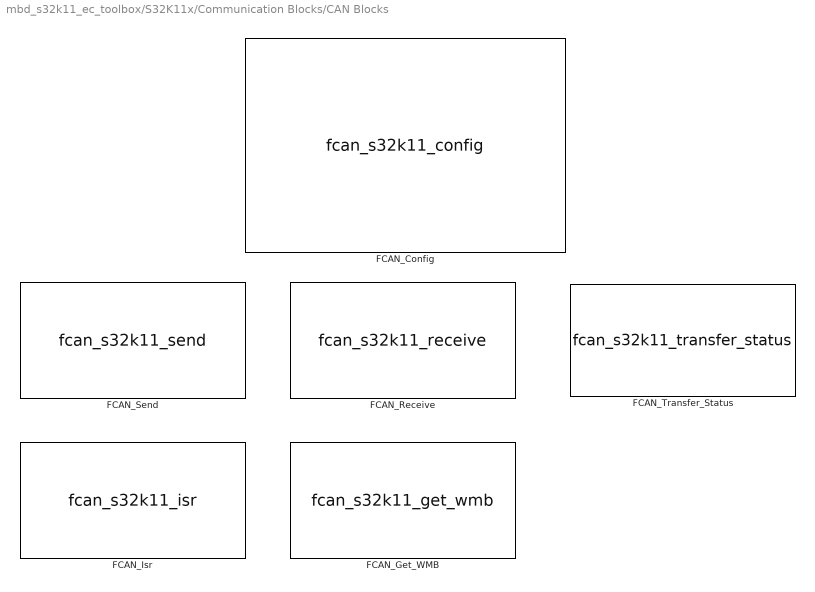
== system mbd_s32k11_ec_toolbox/S32K11x/Communication Blocks/CAN Blocks ==
  FCAN_Config : S-Function  FunctionName=fcan_s32k11_config  SFunctionDeploymentMode=off  EnableBusSupport=off  mask(fcan_s32k11_config){can_instance=0, can_mode=Normal mode, can_max_num_mb=0, can_rx=PTE4: [CAN0_RX | CAN Rx channel], can_tx=PTE5: [CAN0_TX | CAN Tx Channel], show_adv_opts=off, can_clk_src=Peripheral clock, bitrate=500, bitrate_adv_opts=off, can_presdiv=3, can_rjw=3, can_pseg1=6, can_pseg2=3, can_propseg=7, can_cbt_presdiv=1, can_cbt_rjw=3, can_cbt_pseg1=7, can_cbt_pseg2=7, can_cbt_propseg=6, can_fd_enable=off, can_payload=8, can_rxfifo_enable=off, can_fifo_id_filter_extended=off, can_fifo_id_filter_remote=off, can_num_id_filters=8, can_fifo_id_format=A, can_fifo_id_filter={'0x0', '0x0', '0x0', '0x0', '0x0', '0x0', '0x0', '0x0'}, can_pn_enable=off, can_wakeup_match=off, can_wakeup_timeout=off, can_timeout_en=off, can_match_timeout=1, can_multiple_matches_en=off, can_num_matches=1, can_idfilter_extendedid=off, can_idfilter_remoteframe=off, can_idfilter_type=Match exact, can_idfilter_id1=0, can_idfilter_id2=0, can_payloadfilter_enable=off, can_payloadfilter_dlclow=0, can_payloadfilter_dlchigh=0, can_payloadfilter_type=Match exact, can_payloadfilter_payload1_b0=0, can_payloadfilter_payload1_b1=0, can_payloadfilter_payload1_b2=0, can_payloadfilter_payload1_b3=0, can_payloadfilter_payload1_b4=0, can_payloadfilter_payload1_b5=0, can_payloadfilter_payload1_b6=0, can_payloadfilter_payload1_b7=0, can_payloadfilter_payload2_b0=0, can_payloadfilter_payload2_b1=0, can_payloadfilter_payload2_b2=0, can_payloadfilter_payload2_b3=0, can_payloadfilter_payload2_b4=0, can_payloadfilter_payload2_b5=0, can_payloadfilter_payload2_b6=0, can_payloadfilter_payload2_b7=0}
      mask prompts: can_instance "CAN Bus"; can_mode "Operational Mode"; can_max_num_mb "Max number of MBs (0 - 32)"; can_rx "Rx:"; can_tx "Tx:"; show_adv_opts "Show advanced options"; can_clk_src "CAN Engine Clock Source"; bitrate "Bitrate(Kbit/s)"; bitrate_adv_opts "Advanced options"; can_presdiv "Prescaler Divider (0-255)"; can_rjw "Resync Jump Width"; can_pseg1 "Phase Segment 1"; can_pseg2 "Phase Segment 2"; can_propseg "Propagation Segment"; can_cbt_presdiv "Prescaler Divider (0-1023)"; can_cbt_rjw "Resync Jump Width"; can_cbt_pseg1 "Phase Segment 1"; can_cbt_pseg2 "Phase Segment 2"; can_cbt_propseg "Propagation Segment"; can_fd_enable "Enable CAN FD"; can_payload "Payload size"; can_rxfifo_enable "Enable Rx FIFO"; can_fifo_id_filter_extended "Extended ID"; can_fifo_id_filter_remote "Remote frame"; can_num_id_filters "Num ID filters"; can_fifo_id_format "ID format"; can_fifo_id_filter "Filter table"; can_pn_enable "Enable Pretended Networking"; can_wakeup_match "Match event"; can_wakeup_timeout "Timeout event"; can_timeout_en "Enable timeout"; can_match_timeout "Timeout (1 - 65535)"; can_multiple_matches_en "Enable multiple matches"; can_num_matches "Needed matches (1 - 255)"; can_idfilter_extendedid "Extended ID"; can_idfilter_remoteframe "Remote frame"; can_idfilter_type "ID filter type"; can_idfilter_id1 "ID value"; can_idfilter_id2 "ID mask"; can_payloadfilter_enable "Enable payload filtering"; can_payloadfilter_dlclow "Min payload size (0 - 8)"; can_payloadfilter_dlchigh "Max payload size (0 - 8)"; can_payloadfilter_type "Payload filter type"; can_payloadfilter_payload1_b0 "B0"; can_payloadfilter_payload1_b1 "B1"; can_payloadfilter_payload1_b2 "B2"; can_payloadfilter_payload1_b3 "B3"; can_payloadfilter_payload1_b4 "B4"; can_payloadfilter_payload1_b5 "B5"; can_payloadfilter_payload1_b6 "B6"; can_payloadfilter_payload1_b7 "B7"; can_payloadfilter_payload2_b0 "B0"; can_payloadfilter_payload2_b1 "B1"; can_payloadfilter_payload2_b2 "B2"; can_payloadfilter_payload2_b3 "B3"; can_payloadfilter_payload2_b4 "B4"; can_payloadfilter_payload2_b5 "B5"; can_payloadfilter_payload2_b6 "B6"; can_payloadfilter_payload2_b7 "B7"
      mask help: This block is allow to configure FlexCAN module.
      mask init:
      | mbd_s32k_fcan_config_init;
      settings: NameChangeFcn=mbd_s32k_name_check (gcb);
      mask Help: web(fullfile(mbd_s32k11_block_help, 'fcan', 'fcan_config.html'));
      mask TypeOptions can_instance: 0
      mask Callback can_instance:
      | mbd_s32k_fcan_config_cbk('can_instance');
      | mbd_s32k_fcan_display_instances();
      mask TypeOptions can_mode: Normal mode | Listen-only mode | Loop-back mode
      mask Callback can_max_num_mb: mbd_s32k_fcan_config_cbk('can_max_num_mb');
      mask TypeOptions can_rx: PTB0: [CAN0_RX | CAN Rx channel] | PTC2: [CAN0_RX | CAN Rx channel] | PTE4: [CAN0_RX | CAN Rx channel]
      mask TypeOptions can_tx: PTB1: [CAN0_TX | CAN Tx Channel] | PTC3: [CAN0_TX | CAN Tx Channel] | PTE5: [CAN0_TX | CAN Tx Channel]
      mask Callback show_adv_opts: mbd_s32k_fcan_config_cbk('show_adv_opts');
      mask TypeOptions can_clk_src: Oscillator clock | Peripheral clock
      mask Callback can_clk_src: mbd_s32k_fcan_config_cbk('can_clk_src')
      mask TypeOptions bitrate: 50 | 100 | 125 | 250 | 500 | 1000
      mask Callback bitrate: mbd_s32k_fcan_config_cbk('bitrate')
      mask Callback bitrate_adv_opts: mbd_s32k_fcan_config_cbk('bitrate_adv_opts')
      mask TypeOptions can_rjw: 0 | 1 | 2 | 3
      mask TypeOptions can_pseg1: 0 | 1 | 2 | 3 | 4 | 5 | 6 | 7
      mask TypeOptions can_pseg2: 1 | 2 | 3 | 4 | 5 | 6 | 7
      mask TypeOptions can_propseg: 0 | 1 | 2 | 3 | 4 | 5 | 6 | 7
      mask TypeOptions can_cbt_rjw: 0 | 1 | 2 | 3
      mask TypeOptions can_cbt_pseg1: 0 | 1 | 2 | 3 | 4 | 5 | 6 | 7
      mask TypeOptions can_cbt_pseg2: 1 | 2 | 3 | 4 | 5 | 6 | 7
      mask TypeOptions can_cbt_propseg: 0 | 1 | 2 | 3 | 4 | 5 | 6 | 7 | 8 | 9 | 10 | 11 | 12 | 13 | 14 | 15 | 16 | 17 | 18 | 19 | 20 | 21 | 22 | 23 | 24 | 25 | 26 | 27 | 28 | 29 | 30 | 31
      mask Callback can_fd_enable: mbd_s32k_fcan_config_cbk('can_fd_enable');
      mask TypeOptions can_payload: 8
      mask Callback can_rxfifo_enable: mbd_s32k_fcan_config_cbk('can_rxfifo_enable');
      mask TypeOptions can_num_id_filters: 8 | 16 | 24 | 32 | 40 | 48 | 56 | 64 | 72 | 80 | 88 | 96 | 104 | 112 | 120 | 128
      mask TypeOptions can_fifo_id_format: A | B | C | D
      mask Callback can_pn_enable: mbd_s32k_fcan_config_cbk('can_pn_enable');
      mask Callback can_timeout_en: mbd_s32k_fcan_config_cbk('can_timeout_en');
      mask Callback can_multiple_matches_en: mbd_s32k_fcan_config_cbk('can_multiple_matches_en');
      mask TypeOptions can_idfilter_type: Match exact | Match greater than or equal to | Match less than or equal to | Match in range
      mask Callback can_payloadfilter_enable: mbd_s32k_fcan_config_cbk('can_payloadfilter_enable');
      mask TypeOptions can_payloadfilter_type: Match exact | Match greater than or equal to | Match less than or equal to | Match in range
      mask DialogControl PinsGroupbox Prompt: Pins
      mask DialogControl CanStandardFrameGroupbox Prompt: CAN Standard Frame
      mask DialogControl ArbitrationPhaseGroupbox Prompt: Arbitration Phase
      mask DialogControl DataPhaseGroupbox Prompt: Data Phase
      mask DialogControl RxFifoFilteringGroupbox Prompt: Rx FIFO Filtering
      mask DialogControl WakeUpEventsGroupbox Prompt: Wake Up Events
      mask DialogControl IdFilteringGroupbox Prompt: ID Filtering
      mask DialogControl PayloadFilteringGroupbox Prompt: Payload Filtering
      mask DialogControl PayloadValueGroupbox Prompt: Payload value
      mask DialogControl PayloadMaskGroupbox Prompt: Payload mask
      mask Display: disp(st);
  FCAN_Get_WMB : S-Function  FunctionName=fcan_s32k11_get_wmb  SFunctionDeploymentMode=off  EnableBusSupport=off  mask(fcan_s32k11_get_wmb){can_instance=0, can_wmb_idx=0}
      mask prompts: can_instance "CAN Bus"; can_wmb_idx "Wake up Message Buffer"
      mask help: This block allows user to get the Rx data received when FlexCAN is in Pretended Networking mode.
      mask init:
      | crlf = sprintf('\n');
      | 
      | st = [
      |     'FCAN Module : ' get_param(gcb, 'can_instance') crlf ...
      |     'Wake up Message Buffer : ' get_param(gcb, 'can_wmb_idx') crlf];
      | 
      | sFuncParams = []';
      settings: NameChangeFcn=mbd_s32k_name_check (gcb);
      mask Help: web(fullfile(mbd_s32k11_block_help, 'fcan', 'fcan_get_wmb.html'));
      mask TypeOptions can_instance: 0
      mask TypeOptions can_wmb_idx: 0 | 1 | 2 | 3
      mask Display:
      | disp(st);
      | 
      | port_label('output', 1, 'ID');
      | port_label('output', 2, 'Data');
      | port_label('output', 3, 'Length');
  FCAN_Isr : S-Function  FunctionName=fcan_s32k11_isr  Parameters=sFuncParams  SFunctionDeploymentMode=off  EnableBusSupport=off  mask(fcan_s32k11_isr){can_instance=0, can_event=Rx Complete}
      mask prompts: can_instance "CAN Bus"; can_event "Event"
      mask help: This block allows to call user function on different FlexCAN events.
      mask init:
      | [maskStr, sFuncParams] = mbd_s32k_fcan_isr();
      settings: NameChangeFcn=mbd_s32k_name_check (gcb);
      mask Help: web(fullfile(mbd_s32k11_block_help, 'fcan', 'fcan_isr.html'));
      mask TypeOptions can_instance: 0
      mask Callback can_instance:
      | mbd_s32k_fcan_isr_cbk('can_instance');
      | mbd_s32k_fcan_display_instances();
      mask TypeOptions can_event: Rx Complete | Rx FIFO Complete | Tx Complete | Wake Up Timeout | Wake Up Match | Rx FIFO Warning | Rx FIFO Overflow
      mask Display:
      | disp(maskStr);
      | 
      | event = get_param(gcb, 'can_event');
      | 
      | rxCompleteEvent = strcmp(event, 'Rx Complete');
      | rxFifoCompleteEvent = strcmp(event, 'Rx FIFO Complete');
      | txComplete = strcmp(event, 'Tx Complete');
      | 
      | port_label('output', 1, 'Trigger');
      | 
      | switch event
      |     case 'Rx Complete'
      |         port_label('output', 2, 'MB Index');
      |         port_label('output', 3, 'ID');
      |         port_label('output', 4, 'Data');
      |         port_label('output', 5, 'Length');
      |         port_label('output', 6, 'Timestamp');
      |     case 'Rx FIFO Complete'
      |         port_label('output', 2, 'ID');
      |         port_label('output', 3, 'Data');
      |         port_label('output', 4, 'Length');
      |         port_label('output', 5, 'Timestamp');
      |     case 'Tx Complete'
      |         port_label('output', 2, 'MB Index');
      |     case 'Rx FIFO Warning'
      |         port_label('output', 2, 'MB Index');
      |     case 'Rx FIFO Overflow'
      |         port_label('output', 2, 'MB Index');
      | end
  FCAN_Receive : S-Function  FunctionName=fcan_s32k11_receive  Parameters=sFuncParams  SFunctionDeploymentMode=off  EnableBusSupport=off  mask(fcan_s32k11_receive){can_instance=0, can_mode=Non-blocking, can_timeout_ms=0, can_mb_idx=0, can_extended_id=off, can_is_remote=off, can_id=0, can_msg_mask=0, show_adv_opts=off, can_use_rxfifo=off, can_fd_enable=off}
      mask prompts: can_instance "CAN Bus"; can_mode "Mode"; can_timeout_ms "Timeout (ms)"; can_mb_idx "Message Buffer"; can_extended_id "Extended ID"; can_is_remote "Remote message"; can_id "ID (0 - 0x7FF)"; can_msg_mask "Message ID mask (0 - 0xFFFFFFFF)"; show_adv_opts "Show advanced options"; can_use_rxfifo "Use Rx FIFO"; can_fd_enable "Enable CAN FD"
      mask help: This block allows the user to receive data throught CAN interface.
      mask init:
      | [maskStr sFuncParams] = mbd_s32k_fcan_receive();
      settings: NameChangeFcn=mbd_s32k_name_check (gcb);
      mask Help: web(fullfile(mbd_s32k11_block_help, 'fcan', 'fcan_receive.html'));
      mask TypeOptions can_instance: 0 | 1 | 2
      mask Callback can_instance: mbd_s32k_fcan_receive_cbk('can_instance');
      mask TypeOptions can_mode: Blocking | Non-blocking
      mask Callback can_mode: mbd_s32k_fcan_receive_cbk('can_mode');
      mask TypeOptions can_mb_idx: 0 | 1 | 2 | 3 | 4 | 5 | 6 | 7 | 8 | 9 | 10 | 11 | 12 | 13 | 14 | 15 | 16 | 17 | 18 | 19 | 20 | 21 | 22 | 23 | 24 | 25 | 26 | 27 | 28 | 29 | 30 | 31
      mask Callback can_extended_id: mbd_s32k_fcan_receive_cbk('can_extended_id');
      mask Callback can_id: mbd_s32k_fcan_receive_cbk('can_id');
      mask Callback can_msg_mask: mbd_s32k_fcan_receive_cbk('can_msg_mask');
      mask Callback show_adv_opts: mbd_s32k_fcan_receive_cbk('show_adv_opts');
      mask Callback can_use_rxfifo: mbd_s32k_fcan_receive_cbk('can_use_rxfifo');
      mask Callback can_fd_enable: mbd_s32k_fcan_receive_cbk('can_fd_enable');
      mask DialogControl MailboxGroupbox Prompt: Mailbox
      mask Display:
      | disp(maskStr);
      | 
      | mode = get_param(gcb, 'can_mode');
      | if strcmp(mode, 'Blocking')
      |     port_label('output', 1, 'Status');
      |     port_label('output', 2, 'ID');
      |     port_label('output', 3, 'Data');
      |     port_label('output', 4, 'Length');
      |     port_label('output', 5, 'Timestamp');
      | end
  FCAN_Send : S-Function  FunctionName=fcan_s32k11_send  Parameters=out  SFunctionDeploymentMode=off  EnableBusSupport=off  mask(fcan_s32k11_send){can_instance=0, can_mode=Non-blocking, can_timeout_ms=0, can_mb_idx=0, can_extended_id=off, can_is_remote=off, can_id=0, show_adv_opts=off, can_fd_enable=off, can_enable_brs=off, can_fd_padding=0}
      mask prompts: can_instance "CAN Bus"; can_mode "Mode"; can_timeout_ms "Timeout (ms)"; can_mb_idx "Message Buffer"; can_extended_id "Extended ID"; can_is_remote "Remote message"; can_id "ID (0 - 0x7FF)"; show_adv_opts "Show advanced options"; can_fd_enable "Enable CAN FD"; can_enable_brs "Enable Bit Rate Switch (BRS)"; can_fd_padding "CAN FD Padding (0 - 0xFF)"
      mask help: This block allows user to send data throught CAN interface.
      mask init:
      | mbd_s32k_fcan_send_init;
      settings: NameChangeFcn=mbd_s32k_name_check (gcb);
      mask Help: web(fullfile(mbd_s32k11_block_help, 'fcan', 'fcan_send.html'));
      mask TypeOptions can_instance: 0 | 1 | 2
      mask Callback can_instance: mbd_s32k_fcan_send_cbk('can_instance');
      mask TypeOptions can_mode: Blocking | Non-blocking
      mask Callback can_mode: mbd_s32k_fcan_send_cbk('can_mode');
      mask TypeOptions can_mb_idx: 0 | 1 | 2 | 3 | 4 | 5 | 6 | 7 | 8 | 9 | 10 | 11 | 12 | 13 | 14 | 15 | 16 | 17 | 18 | 19 | 20 | 21 | 22 | 23 | 24 | 25 | 26 | 27 | 28 | 29 | 30 | 31
      mask Callback can_extended_id: mbd_s32k_fcan_send_cbk('can_extended_id');
      mask Callback can_id: mbd_s32k_fcan_send_cbk('can_id');
      mask Callback show_adv_opts: mbd_s32k_fcan_send_cbk('show_adv_opts');
      mask Callback can_fd_enable: mbd_s32k_fcan_send_cbk('can_fd_enable');
      mask Callback can_fd_padding: mbd_s32k_fcan_send_cbk('can_fd_padding');
      mask DialogControl MailboxGroupbox Prompt: Mailbox
      mask DialogControl CanFdGroupbox Prompt: CAN FD
      mask Display:
      | disp(st);
      | 
      | port_label('input', 1, 'Data');
      | port_label('input', 2, 'Length');
      | 
      | mode = get_param(gcb, 'can_mode');
      | if strcmp(mode, 'Blocking')
      |     port_label('output', 1, 'Status');
      | end
  FCAN_Transfer_Status : S-Function  FunctionName=fcan_s32k11_transfer_status  SFunctionDeploymentMode=off  EnableBusSupport=off  mask(fcan_s32k11_transfer_status){can_instance=0, can_mb_idx=0}
      mask prompts: can_instance "CAN Bus"; can_mb_idx "Message Buffer"
      mask help: This block allows the user to query if a FlexCAN transfer has finished.
      mask init:
      | mbd_s32k_fcan_transfer_status_init;
      settings: NameChangeFcn=mbd_s32k_name_check (gcb);
      mask Help: web(fullfile(mbd_s32k11_block_help, 'fcan', 'fcan_transfer_status.html'));
      mask TypeOptions can_instance: 0 | 1 | 2
      mask Callback can_instance: mbd_s32k_fcan_transfer_status_cbk('can_instance');
      mask TypeOptions can_mb_idx: 0 | 1 | 2 | 3 | 4 | 5 | 6 | 7 | 8 | 9 | 10 | 11 | 12 | 13 | 14 | 15 | 16 | 17 | 18 | 19 | 20 | 21 | 22 | 23 | 24 | 25 | 26 | 27 | 28 | 29 | 30 | 31
      mask Display:
      | disp(st);
      | 
      | port_label('output', 1, 'Busy');
